simulink model "MMADC"  (R2021a)
settings: Solver=VariableStepAuto  StartTime=0.0  StopTime=1  RelTol=1e-3
values from neighbouring files (symbols this model uses):
  Cf = minimum_cap    [MMADC_main.m]
  clk_freq = 2.1*(nb_MAC+1)/nb_MAC*input_BW    (= 1684.375)    [MMADC_main.m]
  clk_period = 1/clk_freq    (= 0.000593692022263)    [MMADC_main.m]
  comparator_high_offset = 0.2*10e-4    (= 0.0002)    [MMADC_main.m]
  comparator_low_offset = -.1*10e-4    (= -0.0001)    [MMADC_main.m]
  comparator_noise_on = noise_on    (= 1)    [MMADC_main.m]
  comparator_noise_rms = 1*k*T* 2/3 / minimum_cap    [MMADC_main.m]
  comparator_offset_on = noise_on    (= 1)    [MMADC_main.m]
  k = 1.38064852e-23    [MMADC_main.m]
  LNA_bandwidth = 2.5*input_BW    (= 2000)    [MMADC_main.m]
  LNA_gain = 10^(36/20)*12*1.5849    (= 1200.00515432)    [MMADC_main.m]
  LNA_input_referred_noise = sqrt(pi/2*LNA_bandwidth*(194*10^-9)^2)    [MMADC_main.m]
  LNA_noise_on = noise_on    (= 1)    [MMADC_main.m]
  MM_incomplete_transfer_coeff = C1/(C1+C2)    [MMADC_main.m]
  MM_leakage_per_clk_cycle = 1    [MMADC_main.m]
  MM_sampling_noise = noise_on*((k*T * C1/(C1+C2)^2) + (k*T*(C1*C2/(C1+C2))/C2^2))    [MMADC_main.m]
  nb_MAC = 384    [MMADC_main.m]
  number_of_bits = 6    [MMADC_main.m]
  sample_time_jitter = 16e-12    (= 1.6e-11)    [MMADC_main.m]
  sampling_gain = Cs/Cf    [MMADC_main.m]
  sampling_jitter_on = noise_on    (= 1)    [MMADC_main.m]
  sensing_matrix = sensing_matrix_large(j:j+min(19,i-1),:)    [MMADC_main.m]
  sim_number = 0    [MMADC_main.m]
  switch_noise_on = noise_on    (= 1)    [MMADC_main.m]
  switching_noise = k*T/Cf    [MMADC_main.m]
  T = 293    [MMADC_main.m]
  Vref = 2    [MMADC_main.m]
  ZOH_delta = 0*Vref/(2^number_of_bits)    (= 0)    [MMADC_main.m]
libraries: simulink x100, simulink_extras x41, dspsigops x21, dspsrcs4 x21, spsFirstOrderFilterLib x1, dspswit3 x1
(part 6 of 10)

== system MMADC/Sensing Channel 8/SAR/ZOH+comparator ==
  Signal in : Inport
  DAC in : Inport  Port=2
  Input : Inport  Port=3
  Clk : Inport  Port=4
  AND{,1..3} (4 alike) : Logic  IconShape=distinctive  AllPortsSameDT=off  OutDataTypeStr=boolean
  Add : Sum  Inputs=+-
  Comparator : Subsystem  TreatAsAtomicUnit=on
      mask Display: text(.5, .5, 'Comparator', 'horizontalAlignment', 'center', 'verticalAlignment', 'middle')
  Compare To Constant : simulink/Logic and Bit Operations/Compare To Constant  relop===  const=2.0  OutDataTypeStr=boolean
  Constant : Constant  Value=ZOH_delta
  Count ZOH's : Subsystem
  D Latch : simulink_extras/Flip Flops/D Latch
      settings: SourceProductBaseCode=SL
  Delay : Delay
  Delay1 : Delay
  MATLAB Function : MATLAB Function  TreatAsAtomicUnit=on
  Multiport Switch : MultiPortSwitch
  Multiport Switch1 : MultiPortSwitch  Inputs=2  DiagnosticForDefault=None
  NOT1 : Logic  Operator=NOT  IconShape=distinctive  AllPortsSameDT=off  OutDataTypeStr=boolean
  OR1 : Logic  Operator=OR  IconShape=distinctive  AllPortsSameDT=off  OutDataTypeStr=boolean
  Old parallel ZOH comparator : Subsystem  Commented=on
      settings: PortSchema="{\"entries\":[{\"content\":{\"sides\":[{\"content\":{\"connectorIds\":[\"In1\",\"In2\"]},\"type\":\"ConnectorPlacement.EquallySpacedRectSide\",\"uuid\":\"06f7f8f5-dbcc-499c-adfd-56368a53e82b\"},{\"content\":{\"connectorIds\":[\"Out1\",\"Out2\"],\"side\":\"RIGHT\"},\"type\":\"ConnectorPlacement.EquallySpacedRectSide\",\"uuid\":\"5c800770-44b8-4ade-ac9f-191ddf2e034d\"},{\"content\":{\"connectorIds\":[\"In3\",\"In4\"],\"side\":\"TOP\"},\"type\":\"ConnectorPlacement.EquallySpacedRectSide\",\"uuid\":\"3f75a154-aff0-4c2f-90be-ad8d6219778d\"},{\"content\":{\"connectorIds\":[\"Out3\"],\"side\":\"BOTTOM\"},\"type\":\"ConnectorPlacement.EquallySpacedRectSide\",\"uuid\":\"1ea40a8b-dc4d-41fb-8cb2-c53fbb8e1a30\"},{\"content\":{\"connectorIds\":[],\"side\":\"HIDDEN\"},\"type\":\"ConnectorPlacement.EquallySpacedRectSide\",\"uuid\":\"dfb5a5fc-2880-46b8-8362-64f780de510f\"}]},\"type\":\"ConnectorPlacement.EquallySpacedConnector\",\"uuid\":\"ce700ed4-f915-4d6f-ac1f-aa4363807448\"}],\"packageUris\":[\"http://schema.mathworks.com/mf0/Connector/R2020b\"],\"version\":\"1.0\"}"
      mask Display: text(.5, .5, 'ZOH comparator', 'horizontalAlignment', 'center', 'verticalAlignment', 'middle')
  Subtract : Sum  Inputs=-+
  Output2 : Outport
  Output1 : Outport  Port=2
  Output : Outport  Port=3
  wires:
  Delay/1 -> Delay1/1, AND3/2
  Constant/1 -> Multiport Switch1/3
  DAC in/1 -> Multiport Switch/2, Subtract/2, Add/2
  D Latch/1 -> AND/1, Output1/1
  Add/1 -> Multiport Switch/3
  Signal in/1 -> Subtract/1, Add/1, Multiport Switch1/2
  Multiport Switch1/1 -> Comparator/1(y(t))
  Comparator/1(Comparator_out) -> Delay/1, AND2/2, Output2/1, NOT1/1
  Delay1/1 -> AND2/1
  MATLAB Function/1(y) -> Multiport Switch1/1, Multiport Switch/1
  Input/1 -> Compare To Constant/1, MATLAB Function/1(SAR_clk_cycle)
  Compare To Constant/1 -> AND1/1
  Count ZOH's/1(Out1) -> Output/1
  Multiport Switch/1 -> Comparator/2(DAC_in)
  OR1/1 -> D Latch/1
  Subtract/1 -> Multiport Switch/4
  NOT1/1 -> AND3/1
  AND3/1 -> OR1/2
  AND2/1 -> OR1/1
  AND/1 -> Count ZOH's/Trigger
  Clk/1 -> AND1/2
  AND1/1 -> D Latch/2, AND/2

== system MMADC/Sensing Channel 8/Sample&hold/Sample switch noise ==
  Input : Inport
  Trigger : TriggerPort  VariantControl=Variant
  Add1 : Sum
  Constant : Constant  Value=sampling_gain
  Constant1 : Constant  Value=0
  Constant2 : Constant  Value=switch_noise_on
  Multiply1 : Gain  Gain=sqrt(k*T/(sampling_gain*Cf))  OutDataTypeStr=Inherit: Same as input
  Product1 : Product
  Product2 : Product
  Random Number1 : RandomNumber  Variance=switching_noise
  Switch : Switch  Criteria=u2 > Threshold
  Zero-Order Hold1 : ZeroOrderHold  SampleTime=-1
  y(t) : Outport
  wires:
  Product2/1 -> y(t)/1
  Random Number1/1 -> Zero-Order Hold1/1
  Multiply1/1 -> Product1/1
  Add1/1 -> Product2/2
  Constant/1 -> Product2/1, Multiply1/1
  Constant2/1 -> Switch/2
  Constant1/1 -> Switch/3
  Product1/1 -> Switch/1
  Zero-Order Hold1/1 -> Product1/2
  Switch/1 -> Add1/1
  Input/1 -> Add1/2

== system MMADC/Sensing Channel 8/Sample&hold/Sample time jitter ==
  x(t) : Inport
  Add : Sum
  Constant : Constant  Value=sampling_jitter_on
  Derivative : Derivative
  Multiply : Gain  Gain=sample_time_jitter
  Product : Product
  Random Number : RandomNumber  SampleTime=clk_period*(number_of_bits+1)
  Switch : Switch  Criteria=u2 > Threshold
  Zero-Order Hold : ZeroOrderHold  SampleTime=-1
  Output : Outport
  wires:
  Random Number/1 -> Zero-Order Hold/1
  x(t)/1 -> Add/1, Switch/3, Derivative/1
  Zero-Order Hold/1 -> Multiply/1
  Product/1 -> Add/2
  Derivative/1 -> Product/1
  Multiply/1 -> Product/2
  Switch/1 -> Output/1
  Add/1 -> Switch/1
  Constant/1 -> Switch/2

== system MMADC/Sensing Channel 8/Subsystem2/Subsystem ==
  In1 : Inport
  In2 : Inport  Port=2
  Switch : Switch  Criteria=u2 ~= 0
  Zero : Constant  Value=0  OutDataTypeStr=Inherit: Inherit via back propagation
  Out1 : Outport
  wires:
  Switch/1 -> Out1/1
  In2/1 -> Switch/3
  In1/1 -> Switch/2
  Zero/1 -> Switch/1

== system MMADC/Sensing Channel 9/SAR/DAC ==
  NOB : Inport
  Vref : Inport  Port=2
  Input_code : Inport  Port=3
  DAC : MATLAB Function  TreatAsAtomicUnit=on
  y : Outport
  wires:
  NOB/1 -> DAC/2(number_of_bits)
  Vref/1 -> DAC/3(Vref)
  DAC/1(out) -> y/1
  Input_code/1 -> DAC/1(input_code)

== system MMADC/Sensing Channel 9/SAR/SAR ==
  Comparator_in : Inport  LatchByDelayingOutsideSignal=on
  ZOH : Inport  Port=2  LatchByDelayingOutsideSignal=on
  Number of bits : Inport  Port=3
  Trigger : TriggerPort  VariantControl=Variant
  SAR : MATLAB Function  TreatAsAtomicUnit=on
  Unit Delay : UnitDelay  SampleTime=-1  HasFrameUpgradeWarning=on
  Unit Delay1 : UnitDelay  SampleTime=-1  HasFrameUpgradeWarning=on
  Output : Outport
  SAR_done : Outport  Port=2  InitialOutput=0
  Output_code : Outport  Port=3  InitialOutput=zeros(number_of_bits, 1)
      settings: VarSizeSig=Yes
  wires:
  Number of bits/1 -> SAR/4(number_of_bits)
  Comparator_in/1 -> SAR/3(comparator_in)
  Unit Delay1/1 -> SAR/2(cycle_in)
  SAR/3(output_code) -> Output_code/1
  Unit Delay/1 -> SAR/1(input_code_decimal)
  SAR/1(output_code_decimal) -> Unit Delay/1
  SAR/4(done) -> SAR_done/1
  ZOH/1 -> SAR/5(ZOH_true)
  SAR/2(cycle_out) -> Output/1, Unit Delay1/1

== system MMADC/Sensing Channel 9/SAR/ZOH+comparator ==
  Signal in : Inport
  DAC in : Inport  Port=2
  Input : Inport  Port=3
  Clk : Inport  Port=4
  AND{,1..3} (4 alike) : Logic  IconShape=distinctive  AllPortsSameDT=off  OutDataTypeStr=boolean
  Add : Sum  Inputs=+-
  Comparator : Subsystem  TreatAsAtomicUnit=on
      mask Display: text(.5, .5, 'Comparator', 'horizontalAlignment', 'center', 'verticalAlignment', 'middle')
  Compare To Constant : simulink/Logic and Bit Operations/Compare To Constant  relop===  const=2.0  OutDataTypeStr=boolean
  Constant : Constant  Value=ZOH_delta
  Count ZOH's : Subsystem
  D Latch : simulink_extras/Flip Flops/D Latch
      settings: SourceProductBaseCode=SL
  Delay : Delay
  Delay1 : Delay
  MATLAB Function : MATLAB Function  TreatAsAtomicUnit=on
  Multiport Switch : MultiPortSwitch
  Multiport Switch1 : MultiPortSwitch  Inputs=2  DiagnosticForDefault=None
  NOT1 : Logic  Operator=NOT  IconShape=distinctive  AllPortsSameDT=off  OutDataTypeStr=boolean
  OR1 : Logic  Operator=OR  IconShape=distinctive  AllPortsSameDT=off  OutDataTypeStr=boolean
  Old parallel ZOH comparator : Subsystem  Commented=on
      settings: PortSchema="{\"entries\":[{\"content\":{\"sides\":[{\"content\":{\"connectorIds\":[\"In1\",\"In2\"]},\"type\":\"ConnectorPlacement.EquallySpacedRectSide\",\"uuid\":\"06f7f8f5-dbcc-499c-adfd-56368a53e82b\"},{\"content\":{\"connectorIds\":[\"Out1\",\"Out2\"],\"side\":\"RIGHT\"},\"type\":\"ConnectorPlacement.EquallySpacedRectSide\",\"uuid\":\"5c800770-44b8-4ade-ac9f-191ddf2e034d\"},{\"content\":{\"connectorIds\":[\"In3\",\"In4\"],\"side\":\"TOP\"},\"type\":\"ConnectorPlacement.EquallySpacedRectSide\",\"uuid\":\"3f75a154-aff0-4c2f-90be-ad8d6219778d\"},{\"content\":{\"connectorIds\":[\"Out3\"],\"side\":\"BOTTOM\"},\"type\":\"ConnectorPlacement.EquallySpacedRectSide\",\"uuid\":\"1ea40a8b-dc4d-41fb-8cb2-c53fbb8e1a30\"},{\"content\":{\"connectorIds\":[],\"side\":\"HIDDEN\"},\"type\":\"ConnectorPlacement.EquallySpacedRectSide\",\"uuid\":\"dfb5a5fc-2880-46b8-8362-64f780de510f\"}]},\"type\":\"ConnectorPlacement.EquallySpacedConnector\",\"uuid\":\"ce700ed4-f915-4d6f-ac1f-aa4363807448\"}],\"packageUris\":[\"http://schema.mathworks.com/mf0/Connector/R2020b\"],\"version\":\"1.0\"}"
      mask Display: text(.5, .5, 'ZOH comparator', 'horizontalAlignment', 'center', 'verticalAlignment', 'middle')
  Subtract : Sum  Inputs=-+
  Output2 : Outport
  Output1 : Outport  Port=2
  Output : Outport  Port=3
  wires:
  Delay/1 -> Delay1/1, AND3/2
  Constant/1 -> Multiport Switch1/3
  DAC in/1 -> Multiport Switch/2, Subtract/2, Add/2
  D Latch/1 -> AND/1, Output1/1
  Add/1 -> Multiport Switch/3
  Signal in/1 -> Subtract/1, Add/1, Multiport Switch1/2
  Multiport Switch1/1 -> Comparator/1(y(t))
  Comparator/1(Comparator_out) -> Delay/1, AND2/2, Output2/1, NOT1/1
  Delay1/1 -> AND2/1
  MATLAB Function/1(y) -> Multiport Switch1/1, Multiport Switch/1
  Input/1 -> Compare To Constant/1, MATLAB Function/1(SAR_clk_cycle)
  Compare To Constant/1 -> AND1/1
  Count ZOH's/1(Out1) -> Output/1
  Multiport Switch/1 -> Comparator/2(DAC_in)
  OR1/1 -> D Latch/1
  Subtract/1 -> Multiport Switch/4
  NOT1/1 -> AND3/1
  AND3/1 -> OR1/2
  AND2/1 -> OR1/1
  AND/1 -> Count ZOH's/Trigger
  Clk/1 -> AND1/2
  AND1/1 -> D Latch/2, AND/2

== system MMADC/Sensing Channel 9/Sample&hold/Sample switch noise ==
  Input : Inport
  Trigger : TriggerPort  VariantControl=Variant
  Add1 : Sum
  Constant : Constant  Value=sampling_gain
  Constant1 : Constant  Value=0
  Constant2 : Constant  Value=switch_noise_on
  Multiply1 : Gain  Gain=sqrt(k*T/(sampling_gain*Cf))  OutDataTypeStr=Inherit: Same as input
  Product1 : Product
  Product2 : Product
  Random Number1 : RandomNumber  Variance=switching_noise
  Switch : Switch  Criteria=u2 > Threshold
  Zero-Order Hold1 : ZeroOrderHold  SampleTime=-1
  y(t) : Outport
  wires:
  Product2/1 -> y(t)/1
  Random Number1/1 -> Zero-Order Hold1/1
  Multiply1/1 -> Product1/1
  Add1/1 -> Product2/2
  Constant/1 -> Product2/1, Multiply1/1
  Constant2/1 -> Switch/2
  Constant1/1 -> Switch/3
  Product1/1 -> Switch/1
  Zero-Order Hold1/1 -> Product1/2
  Switch/1 -> Add1/1
  Input/1 -> Add1/2

== system MMADC/Sensing Channel 9/Sample&hold/Sample time jitter ==
  x(t) : Inport
  Add : Sum
  Constant : Constant  Value=sampling_jitter_on
  Derivative : Derivative
  Multiply : Gain  Gain=sample_time_jitter
  Product : Product
  Random Number : RandomNumber  SampleTime=clk_period*(number_of_bits+1)
  Switch : Switch  Criteria=u2 > Threshold
  Zero-Order Hold : ZeroOrderHold  SampleTime=-1
  Output : Outport
  wires:
  Random Number/1 -> Zero-Order Hold/1
  x(t)/1 -> Add/1, Switch/3, Derivative/1
  Zero-Order Hold/1 -> Multiply/1
  Product/1 -> Add/2
  Derivative/1 -> Product/1
  Multiply/1 -> Product/2
  Switch/1 -> Output/1
  Add/1 -> Switch/1
  Constant/1 -> Switch/2

== system MMADC/Sensing Channel 9/Subsystem2/Subsystem ==
  In1 : Inport
  In2 : Inport  Port=2
  Switch : Switch  Criteria=u2 ~= 0
  Zero : Constant  Value=0  OutDataTypeStr=Inherit: Inherit via back propagation
  Out1 : Outport
  wires:
  Switch/1 -> Out1/1
  In2/1 -> Switch/3
  In1/1 -> Switch/2
  Zero/1 -> Switch/1

== system MMADC/Sensing Channel 1/SAR/ZOH+comparator/Comparator ==
  y(t) : Inport
  DAC_in : Inport  Port=2
  Add : Sum
  Add1 : Sum
  Compare To Zero : simulink/Logic and Bit Operations/Compare To Zero  relop=>  OutDataTypeStr=boolean
  Constant : Constant  Value=comparator_high_offset
  Constant1 : Constant  Value=comparator_low_offset
  Constant2 : Constant  Value=0
  Constant3 : Constant  Value=comparator_offset_on
  Constant4 : Constant  Value=0
  Constant5 : Constant  Value=comparator_noise_on
  Multiply : Gain  Gain=comparator_noise_rms
  Random Number : RandomNumber  Seed=sim_number  SampleTime=1/clk_freq
  Subtract : Sum  Inputs=+-
  Switch : Switch  Criteria=u2 > Threshold
  Switch1 : Switch  Criteria=u2 > Threshold
  Switch2 : Switch  Criteria=u2 > Threshold
  Unit Delay : UnitDelay  SampleTime=-1  HasFrameUpgradeWarning=on
  Comparator_out : Outport
  wires:
  Switch/1 -> Switch1/1
  Subtract/1 -> Add/1
  Constant/1 -> Switch/1
  Constant2/1 -> Switch1/3
  Add/1 -> Compare To Zero/1
  Switch1/1 -> Add/2
  Constant3/1 -> Switch1/2
  Unit Delay/1 -> Switch/2
  Constant1/1 -> Switch/3
  DAC_in/1 -> Subtract/2
  Add1/1 -> Subtract/1
  y(t)/1 -> Add1/2
  Random Number/1 -> Multiply/1
  Switch2/1 -> Add1/1
  Multiply/1 -> Switch2/1
  Constant4/1 -> Switch2/3
  Constant5/1 -> Switch2/2
  Compare To Zero/1 -> Unit Delay/1, Comparator_out/1

== system MMADC/Sensing Channel 1/SAR/ZOH+comparator/Count ZOH's ==
  Trigger : TriggerPort  VariantControl=Variant  PortDimensions=1
  Add : Sum  AccumDataTypeStr=double  OutDataTypeStr=double
  Constant : Constant
  Unit Delay : UnitDelay  SampleTime=-1  HasFrameUpgradeWarning=on
  Out1 : Outport
  wires:
  Constant/1 -> Add/1
  Add/1 -> Unit Delay/1, Out1/1
  Unit Delay/1 -> Add/2

== system MMADC/Sensing Channel 1/SAR/ZOH+comparator/Old parallel ZOH comparator ==
  Signal in : Inport
  DAC in : Inport  Port=2
  SAR done : Inport  Port=3
  Clk : Inport  Port=4
  " DAC-signal < delta?" : Subsystem  TreatAsAtomicUnit=on
      mask Display: text(.5, .5, 'Comparator', 'horizontalAlignment', 'center', 'verticalAlignment', 'middle')
  AND : Logic  IconShape=distinctive  AllPortsSameDT=off  OutDataTypeStr=boolean
  AND1 : Logic  IconShape=distinctive  AllPortsSameDT=off  OutDataTypeStr=boolean
  Add : Sum  Inputs=+-
  Constant : Constant  Value=ZOH_delta
  Count ZOH's : Subsystem
  D Latch : simulink_extras/Flip Flops/D Latch
      settings: SourceProductBaseCode=SL
  NOT : Logic  Operator=NOT  IconShape=distinctive  AllPortsSameDT=off  OutDataTypeStr=boolean
  OR : Logic  Operator=OR  IconShape=distinctive  AllPortsSameDT=off  OutDataTypeStr=boolean
  Signal-DAC < delta? : Subsystem  TreatAsAtomicUnit=on
      mask Display: text(.5, .5, 'Comparator', 'horizontalAlignment', 'center', 'verticalAlignment', 'middle')
  Signal>DAC? : Subsystem  TreatAsAtomicUnit=on
      mask Display: text(.5, .5, 'Comparator', 'horizontalAlignment', 'center', 'verticalAlignment', 'middle')
  Subtract : Sum  Inputs=-+
  Comparator_out : Outport
  Output1 : Outport  Port=2
  Output : Outport  Port=3
  wires:
  Signal>DAC?/1(Comparator_out) -> NOT/1, Comparator_out/1, AND1/1
  AND1/1 -> OR/1
  Subtract/1 -> " DAC-signal < delta?"/2(DAC_in)
  Signal in/1 -> Add/1, Subtract/1, Signal>DAC?/1(y(t))
  Clk/1 -> Signal>DAC?/Trigger, Signal-DAC < delta?/Trigger, " DAC-signal < delta?"/Trigger
  AND/1 -> OR/2
  " DAC-signal < delta?"/1(Comparator_out) -> AND/2  "comp2"
  Signal-DAC < delta?/1(Comparator_out) -> AND1/2  "comp1"
  Add/1 -> Signal-DAC < delta?/2(DAC_in)
  DAC in/1 -> Subtract/2, Add/2, Signal>DAC?/2(DAC_in)
  Constant/1 -> Signal-DAC < delta?/1(y(t)), " DAC-signal < delta?"/1(y(t))
  NOT/1 -> AND/1
  OR/1 -> D Latch/1
  D Latch/1 -> Count ZOH's/1(In1), Output1/1
  Count ZOH's/1(Out1) -> Output/1
  SAR done/1 -> Count ZOH's/Trigger, D Latch/2

== system MMADC/Sensing Channel 10/SAR/ZOH+comparator/Comparator ==
  y(t) : Inport
  DAC_in : Inport  Port=2
  Add : Sum
  Add1 : Sum
  Compare To Zero : simulink/Logic and Bit Operations/Compare To Zero  relop=>  OutDataTypeStr=boolean
  Constant : Constant  Value=comparator_high_offset
  Constant1 : Constant  Value=comparator_low_offset
  Constant2 : Constant  Value=0
  Constant3 : Constant  Value=comparator_offset_on
  Constant4 : Constant  Value=0
  Constant5 : Constant  Value=comparator_noise_on
  Multiply : Gain  Gain=comparator_noise_rms
  Random Number : RandomNumber  SampleTime=1/clk_freq
  Subtract : Sum  Inputs=+-
  Switch : Switch  Criteria=u2 > Threshold
  Switch1 : Switch  Criteria=u2 > Threshold
  Switch2 : Switch  Criteria=u2 > Threshold
  Unit Delay : UnitDelay  SampleTime=-1  HasFrameUpgradeWarning=on
  Comparator_out : Outport
  wires:
  Switch/1 -> Switch1/1
  Subtract/1 -> Add/1
  Constant/1 -> Switch/1
  Constant2/1 -> Switch1/3
  Add/1 -> Compare To Zero/1
  Switch1/1 -> Add/2
  Constant3/1 -> Switch1/2
  Unit Delay/1 -> Switch/2
  Constant1/1 -> Switch/3
  DAC_in/1 -> Subtract/2
  Add1/1 -> Subtract/1
  y(t)/1 -> Add1/2
  Random Number/1 -> Multiply/1
  Switch2/1 -> Add1/1
  Multiply/1 -> Switch2/1
  Constant4/1 -> Switch2/3
  Constant5/1 -> Switch2/2
  Compare To Zero/1 -> Unit Delay/1, Comparator_out/1

== system MMADC/Sensing Channel 10/SAR/ZOH+comparator/Count ZOH's ==
  Trigger : TriggerPort  VariantControl=Variant  PortDimensions=1
  Add : Sum  AccumDataTypeStr=double  OutDataTypeStr=double
  Constant : Constant
  Unit Delay : UnitDelay  SampleTime=-1  HasFrameUpgradeWarning=on
  Out1 : Outport
  wires:
  Constant/1 -> Add/1
  Add/1 -> Unit Delay/1, Out1/1
  Unit Delay/1 -> Add/2

== system MMADC/Sensing Channel 10/SAR/ZOH+comparator/Old parallel ZOH comparator ==
  Signal in : Inport
  DAC in : Inport  Port=2
  SAR done : Inport  Port=3
  Clk : Inport  Port=4
  " DAC-signal < delta?" : Subsystem  TreatAsAtomicUnit=on
      mask Display: text(.5, .5, 'Comparator', 'horizontalAlignment', 'center', 'verticalAlignment', 'middle')
  AND : Logic  IconShape=distinctive  AllPortsSameDT=off  OutDataTypeStr=boolean
  AND1 : Logic  IconShape=distinctive  AllPortsSameDT=off  OutDataTypeStr=boolean
  Add : Sum  Inputs=+-
  Constant : Constant  Value=ZOH_delta
  Count ZOH's : Subsystem
  D Latch : simulink_extras/Flip Flops/D Latch
      settings: SourceProductBaseCode=SL
  NOT : Logic  Operator=NOT  IconShape=distinctive  AllPortsSameDT=off  OutDataTypeStr=boolean
  OR : Logic  Operator=OR  IconShape=distinctive  AllPortsSameDT=off  OutDataTypeStr=boolean
  Signal-DAC < delta? : Subsystem  TreatAsAtomicUnit=on
      mask Display: text(.5, .5, 'Comparator', 'horizontalAlignment', 'center', 'verticalAlignment', 'middle')
  Signal>DAC? : Subsystem  TreatAsAtomicUnit=on
      mask Display: text(.5, .5, 'Comparator', 'horizontalAlignment', 'center', 'verticalAlignment', 'middle')
  Subtract : Sum  Inputs=-+
  Comparator_out : Outport
  Output1 : Outport  Port=2
  Output : Outport  Port=3
  wires:
  Signal>DAC?/1(Comparator_out) -> NOT/1, Comparator_out/1, AND1/1
  AND1/1 -> OR/1
  Subtract/1 -> " DAC-signal < delta?"/2(DAC_in)
  Signal in/1 -> Add/1, Subtract/1, Signal>DAC?/1(y(t))
  Clk/1 -> Signal>DAC?/Trigger, Signal-DAC < delta?/Trigger, " DAC-signal < delta?"/Trigger
  AND/1 -> OR/2
  " DAC-signal < delta?"/1(Comparator_out) -> AND/2  "comp2"
  Signal-DAC < delta?/1(Comparator_out) -> AND1/2  "comp1"
  Add/1 -> Signal-DAC < delta?/2(DAC_in)
  DAC in/1 -> Subtract/2, Add/2, Signal>DAC?/2(DAC_in)
  Constant/1 -> Signal-DAC < delta?/1(y(t)), " DAC-signal < delta?"/1(y(t))
  NOT/1 -> AND/1
  OR/1 -> D Latch/1
  D Latch/1 -> Count ZOH's/1(In1), Output1/1
  Count ZOH's/1(Out1) -> Output/1
  SAR done/1 -> Count ZOH's/Trigger, D Latch/2

== system MMADC/Sensing Channel 11/SAR/ZOH+comparator/Comparator ==
  y(t) : Inport
  DAC_in : Inport  Port=2
  Add : Sum
  Add1 : Sum
  Compare To Zero : simulink/Logic and Bit Operations/Compare To Zero  relop=>  OutDataTypeStr=boolean
  Constant : Constant  Value=comparator_high_offset
  Constant1 : Constant  Value=comparator_low_offset
  Constant2 : Constant  Value=0
  Constant3 : Constant  Value=comparator_offset_on
  Constant4 : Constant  Value=0
  Constant5 : Constant  Value=comparator_noise_on
  Multiply : Gain  Gain=comparator_noise_rms
  Random Number : RandomNumber  SampleTime=1/clk_freq
  Subtract : Sum  Inputs=+-
  Switch : Switch  Criteria=u2 > Threshold
  Switch1 : Switch  Criteria=u2 > Threshold
  Switch2 : Switch  Criteria=u2 > Threshold
  Unit Delay : UnitDelay  SampleTime=-1  HasFrameUpgradeWarning=on
  Comparator_out : Outport
  wires:
  Switch/1 -> Switch1/1
  Subtract/1 -> Add/1
  Constant/1 -> Switch/1
  Constant2/1 -> Switch1/3
  Add/1 -> Compare To Zero/1
  Switch1/1 -> Add/2
  Constant3/1 -> Switch1/2
  Unit Delay/1 -> Switch/2
  Constant1/1 -> Switch/3
  DAC_in/1 -> Subtract/2
  Add1/1 -> Subtract/1
  y(t)/1 -> Add1/2
  Random Number/1 -> Multiply/1
  Switch2/1 -> Add1/1
  Multiply/1 -> Switch2/1
  Constant4/1 -> Switch2/3
  Constant5/1 -> Switch2/2
  Compare To Zero/1 -> Unit Delay/1, Comparator_out/1

== system MMADC/Sensing Channel 11/SAR/ZOH+comparator/Count ZOH's ==
  Trigger : TriggerPort  VariantControl=Variant  PortDimensions=1
  Add : Sum  AccumDataTypeStr=double  OutDataTypeStr=double
  Constant : Constant
  Unit Delay : UnitDelay  SampleTime=-1  HasFrameUpgradeWarning=on
  Out1 : Outport
  wires:
  Constant/1 -> Add/1
  Add/1 -> Unit Delay/1, Out1/1
  Unit Delay/1 -> Add/2

== system MMADC/Sensing Channel 11/SAR/ZOH+comparator/Old parallel ZOH comparator ==
  Signal in : Inport
  DAC in : Inport  Port=2
  SAR done : Inport  Port=3
  Clk : Inport  Port=4
  " DAC-signal < delta?" : Subsystem  TreatAsAtomicUnit=on
      mask Display: text(.5, .5, 'Comparator', 'horizontalAlignment', 'center', 'verticalAlignment', 'middle')
  AND : Logic  IconShape=distinctive  AllPortsSameDT=off  OutDataTypeStr=boolean
  AND1 : Logic  IconShape=distinctive  AllPortsSameDT=off  OutDataTypeStr=boolean
  Add : Sum  Inputs=+-
  Constant : Constant  Value=ZOH_delta
  Count ZOH's : Subsystem
  D Latch : simulink_extras/Flip Flops/D Latch
      settings: SourceProductBaseCode=SL
  NOT : Logic  Operator=NOT  IconShape=distinctive  AllPortsSameDT=off  OutDataTypeStr=boolean
  OR : Logic  Operator=OR  IconShape=distinctive  AllPortsSameDT=off  OutDataTypeStr=boolean
  Signal-DAC < delta? : Subsystem  TreatAsAtomicUnit=on
      mask Display: text(.5, .5, 'Comparator', 'horizontalAlignment', 'center', 'verticalAlignment', 'middle')
  Signal>DAC? : Subsystem  TreatAsAtomicUnit=on
      mask Display: text(.5, .5, 'Comparator', 'horizontalAlignment', 'center', 'verticalAlignment', 'middle')
  Subtract : Sum  Inputs=-+
  Comparator_out : Outport
  Output1 : Outport  Port=2
  Output : Outport  Port=3
  wires:
  Signal>DAC?/1(Comparator_out) -> NOT/1, Comparator_out/1, AND1/1
  AND1/1 -> OR/1
  Subtract/1 -> " DAC-signal < delta?"/2(DAC_in)
  Signal in/1 -> Add/1, Subtract/1, Signal>DAC?/1(y(t))
  Clk/1 -> Signal>DAC?/Trigger, Signal-DAC < delta?/Trigger, " DAC-signal < delta?"/Trigger
  AND/1 -> OR/2
  " DAC-signal < delta?"/1(Comparator_out) -> AND/2  "comp2"
  Signal-DAC < delta?/1(Comparator_out) -> AND1/2  "comp1"
  Add/1 -> Signal-DAC < delta?/2(DAC_in)
  DAC in/1 -> Subtract/2, Add/2, Signal>DAC?/2(DAC_in)
  Constant/1 -> Signal-DAC < delta?/1(y(t)), " DAC-signal < delta?"/1(y(t))
  NOT/1 -> AND/1
  OR/1 -> D Latch/1
  D Latch/1 -> Count ZOH's/1(In1), Output1/1
  Count ZOH's/1(Out1) -> Output/1
  SAR done/1 -> Count ZOH's/Trigger, D Latch/2

== system MMADC/Sensing Channel 12/SAR/ZOH+comparator/Comparator ==
  y(t) : Inport
  DAC_in : Inport  Port=2
  Add : Sum
  Add1 : Sum
  Compare To Zero : simulink/Logic and Bit Operations/Compare To Zero  relop=>  OutDataTypeStr=boolean
  Constant : Constant  Value=comparator_high_offset
  Constant1 : Constant  Value=comparator_low_offset
  Constant2 : Constant  Value=0
  Constant3 : Constant  Value=comparator_offset_on
  Constant4 : Constant  Value=0
  Constant5 : Constant  Value=comparator_noise_on
  Multiply : Gain  Gain=comparator_noise_rms
  Random Number : RandomNumber  SampleTime=1/clk_freq
  Subtract : Sum  Inputs=+-
  Switch : Switch  Criteria=u2 > Threshold
  Switch1 : Switch  Criteria=u2 > Threshold
  Switch2 : Switch  Criteria=u2 > Threshold
  Unit Delay : UnitDelay  SampleTime=-1  HasFrameUpgradeWarning=on
  Comparator_out : Outport
  wires:
  Switch/1 -> Switch1/1
  Subtract/1 -> Add/1
  Constant/1 -> Switch/1
  Constant2/1 -> Switch1/3
  Add/1 -> Compare To Zero/1
  Switch1/1 -> Add/2
  Constant3/1 -> Switch1/2
  Unit Delay/1 -> Switch/2
  Constant1/1 -> Switch/3
  DAC_in/1 -> Subtract/2
  Add1/1 -> Subtract/1
  y(t)/1 -> Add1/2
  Random Number/1 -> Multiply/1
  Switch2/1 -> Add1/1
  Multiply/1 -> Switch2/1
  Constant4/1 -> Switch2/3
  Constant5/1 -> Switch2/2
  Compare To Zero/1 -> Unit Delay/1, Comparator_out/1

== system MMADC/Sensing Channel 12/SAR/ZOH+comparator/Count ZOH's ==
  Trigger : TriggerPort  VariantControl=Variant  PortDimensions=1
  Add : Sum  AccumDataTypeStr=double  OutDataTypeStr=double
  Constant : Constant
  Unit Delay : UnitDelay  SampleTime=-1  HasFrameUpgradeWarning=on
  Out1 : Outport
  wires:
  Constant/1 -> Add/1
  Add/1 -> Unit Delay/1, Out1/1
  Unit Delay/1 -> Add/2

== system MMADC/Sensing Channel 12/SAR/ZOH+comparator/Old parallel ZOH comparator ==
  Signal in : Inport
  DAC in : Inport  Port=2
  SAR done : Inport  Port=3
  Clk : Inport  Port=4
  " DAC-signal < delta?" : Subsystem  TreatAsAtomicUnit=on
      mask Display: text(.5, .5, 'Comparator', 'horizontalAlignment', 'center', 'verticalAlignment', 'middle')
  AND : Logic  IconShape=distinctive  AllPortsSameDT=off  OutDataTypeStr=boolean
  AND1 : Logic  IconShape=distinctive  AllPortsSameDT=off  OutDataTypeStr=boolean
  Add : Sum  Inputs=+-
  Constant : Constant  Value=ZOH_delta
  Count ZOH's : Subsystem
  D Latch : simulink_extras/Flip Flops/D Latch
      settings: SourceProductBaseCode=SL
  NOT : Logic  Operator=NOT  IconShape=distinctive  AllPortsSameDT=off  OutDataTypeStr=boolean
  OR : Logic  Operator=OR  IconShape=distinctive  AllPortsSameDT=off  OutDataTypeStr=boolean
  Signal-DAC < delta? : Subsystem  TreatAsAtomicUnit=on
      mask Display: text(.5, .5, 'Comparator', 'horizontalAlignment', 'center', 'verticalAlignment', 'middle')
  Signal>DAC? : Subsystem  TreatAsAtomicUnit=on
      mask Display: text(.5, .5, 'Comparator', 'horizontalAlignment', 'center', 'verticalAlignment', 'middle')
  Subtract : Sum  Inputs=-+
  Comparator_out : Outport
  Output1 : Outport  Port=2
  Output : Outport  Port=3
  wires:
  Signal>DAC?/1(Comparator_out) -> NOT/1, Comparator_out/1, AND1/1
  AND1/1 -> OR/1
  Subtract/1 -> " DAC-signal < delta?"/2(DAC_in)
  Signal in/1 -> Add/1, Subtract/1, Signal>DAC?/1(y(t))
  Clk/1 -> Signal>DAC?/Trigger, Signal-DAC < delta?/Trigger, " DAC-signal < delta?"/Trigger
  AND/1 -> OR/2
  " DAC-signal < delta?"/1(Comparator_out) -> AND/2  "comp2"
  Signal-DAC < delta?/1(Comparator_out) -> AND1/2  "comp1"
  Add/1 -> Signal-DAC < delta?/2(DAC_in)
  DAC in/1 -> Subtract/2, Add/2, Signal>DAC?/2(DAC_in)
  Constant/1 -> Signal-DAC < delta?/1(y(t)), " DAC-signal < delta?"/1(y(t))
  NOT/1 -> AND/1
  OR/1 -> D Latch/1
  D Latch/1 -> Count ZOH's/1(In1), Output1/1
  Count ZOH's/1(Out1) -> Output/1
  SAR done/1 -> Count ZOH's/Trigger, D Latch/2

== system MMADC/Sensing Channel 13/SAR/ZOH+comparator/Comparator ==
  y(t) : Inport
  DAC_in : Inport  Port=2
  Add : Sum
  Add1 : Sum
  Compare To Zero : simulink/Logic and Bit Operations/Compare To Zero  relop=>  OutDataTypeStr=boolean
  Constant : Constant  Value=comparator_high_offset
  Constant1 : Constant  Value=comparator_low_offset
  Constant2 : Constant  Value=0
  Constant3 : Constant  Value=comparator_offset_on
  Constant4 : Constant  Value=0
  Constant5 : Constant  Value=comparator_noise_on
  Multiply : Gain  Gain=comparator_noise_rms
  Random Number : RandomNumber  SampleTime=1/clk_freq
  Subtract : Sum  Inputs=+-
  Switch : Switch  Criteria=u2 > Threshold
  Switch1 : Switch  Criteria=u2 > Threshold
  Switch2 : Switch  Criteria=u2 > Threshold
  Unit Delay : UnitDelay  SampleTime=-1  HasFrameUpgradeWarning=on
  Comparator_out : Outport
  wires:
  Switch/1 -> Switch1/1
  Subtract/1 -> Add/1
  Constant/1 -> Switch/1
  Constant2/1 -> Switch1/3
  Add/1 -> Compare To Zero/1
  Switch1/1 -> Add/2
  Constant3/1 -> Switch1/2
  Unit Delay/1 -> Switch/2
  Constant1/1 -> Switch/3
  DAC_in/1 -> Subtract/2
  Add1/1 -> Subtract/1
  y(t)/1 -> Add1/2
  Random Number/1 -> Multiply/1
  Switch2/1 -> Add1/1
  Multiply/1 -> Switch2/1
  Constant4/1 -> Switch2/3
  Constant5/1 -> Switch2/2
  Compare To Zero/1 -> Unit Delay/1, Comparator_out/1

== system MMADC/Sensing Channel 13/SAR/ZOH+comparator/Count ZOH's ==
  Trigger : TriggerPort  VariantControl=Variant  PortDimensions=1
  Add : Sum  AccumDataTypeStr=double  OutDataTypeStr=double
  Constant : Constant
  Unit Delay : UnitDelay  SampleTime=-1  HasFrameUpgradeWarning=on
  Out1 : Outport
  wires:
  Constant/1 -> Add/1
  Add/1 -> Unit Delay/1, Out1/1
  Unit Delay/1 -> Add/2

== system MMADC/Sensing Channel 13/SAR/ZOH+comparator/Old parallel ZOH comparator ==
  Signal in : Inport
  DAC in : Inport  Port=2
  SAR done : Inport  Port=3
  Clk : Inport  Port=4
  " DAC-signal < delta?" : Subsystem  TreatAsAtomicUnit=on
      mask Display: text(.5, .5, 'Comparator', 'horizontalAlignment', 'center', 'verticalAlignment', 'middle')
  AND : Logic  IconShape=distinctive  AllPortsSameDT=off  OutDataTypeStr=boolean
  AND1 : Logic  IconShape=distinctive  AllPortsSameDT=off  OutDataTypeStr=boolean
  Add : Sum  Inputs=+-
  Constant : Constant  Value=ZOH_delta
  Count ZOH's : Subsystem
  D Latch : simulink_extras/Flip Flops/D Latch
      settings: SourceProductBaseCode=SL
  NOT : Logic  Operator=NOT  IconShape=distinctive  AllPortsSameDT=off  OutDataTypeStr=boolean
  OR : Logic  Operator=OR  IconShape=distinctive  AllPortsSameDT=off  OutDataTypeStr=boolean
  Signal-DAC < delta? : Subsystem  TreatAsAtomicUnit=on
      mask Display: text(.5, .5, 'Comparator', 'horizontalAlignment', 'center', 'verticalAlignment', 'middle')
  Signal>DAC? : Subsystem  TreatAsAtomicUnit=on
      mask Display: text(.5, .5, 'Comparator', 'horizontalAlignment', 'center', 'verticalAlignment', 'middle')
  Subtract : Sum  Inputs=-+
  Comparator_out : Outport
  Output1 : Outport  Port=2
  Output : Outport  Port=3
  wires:
  Signal>DAC?/1(Comparator_out) -> NOT/1, Comparator_out/1, AND1/1
  AND1/1 -> OR/1
  Subtract/1 -> " DAC-signal < delta?"/2(DAC_in)
  Signal in/1 -> Add/1, Subtract/1, Signal>DAC?/1(y(t))
  Clk/1 -> Signal>DAC?/Trigger, Signal-DAC < delta?/Trigger, " DAC-signal < delta?"/Trigger
  AND/1 -> OR/2
  " DAC-signal < delta?"/1(Comparator_out) -> AND/2  "comp2"
  Signal-DAC < delta?/1(Comparator_out) -> AND1/2  "comp1"
  Add/1 -> Signal-DAC < delta?/2(DAC_in)
  DAC in/1 -> Subtract/2, Add/2, Signal>DAC?/2(DAC_in)
  Constant/1 -> Signal-DAC < delta?/1(y(t)), " DAC-signal < delta?"/1(y(t))
  NOT/1 -> AND/1
  OR/1 -> D Latch/1
  D Latch/1 -> Count ZOH's/1(In1), Output1/1
  Count ZOH's/1(Out1) -> Output/1
  SAR done/1 -> Count ZOH's/Trigger, D Latch/2

== system MMADC/Sensing Channel 14/SAR/ZOH+comparator/Comparator ==
  y(t) : Inport
  DAC_in : Inport  Port=2
  Add : Sum
  Add1 : Sum
  Compare To Zero : simulink/Logic and Bit Operations/Compare To Zero  relop=>  OutDataTypeStr=boolean
  Constant : Constant  Value=comparator_high_offset
  Constant1 : Constant  Value=comparator_low_offset
  Constant2 : Constant  Value=0
  Constant3 : Constant  Value=comparator_offset_on
  Constant4 : Constant  Value=0
  Constant5 : Constant  Value=comparator_noise_on
  Multiply : Gain  Gain=comparator_noise_rms
  Random Number : RandomNumber  SampleTime=1/clk_freq
  Subtract : Sum  Inputs=+-
  Switch : Switch  Criteria=u2 > Threshold
  Switch1 : Switch  Criteria=u2 > Threshold
  Switch2 : Switch  Criteria=u2 > Threshold
  Unit Delay : UnitDelay  SampleTime=-1  HasFrameUpgradeWarning=on
  Comparator_out : Outport
  wires:
  Switch/1 -> Switch1/1
  Subtract/1 -> Add/1
  Constant/1 -> Switch/1
  Constant2/1 -> Switch1/3
  Add/1 -> Compare To Zero/1
  Switch1/1 -> Add/2
  Constant3/1 -> Switch1/2
  Unit Delay/1 -> Switch/2
  Constant1/1 -> Switch/3
  DAC_in/1 -> Subtract/2
  Add1/1 -> Subtract/1
  y(t)/1 -> Add1/2
  Random Number/1 -> Multiply/1
  Switch2/1 -> Add1/1
  Multiply/1 -> Switch2/1
  Constant4/1 -> Switch2/3
  Constant5/1 -> Switch2/2
  Compare To Zero/1 -> Unit Delay/1, Comparator_out/1

== system MMADC/Sensing Channel 14/SAR/ZOH+comparator/Count ZOH's ==
  Trigger : TriggerPort  VariantControl=Variant  PortDimensions=1
  Add : Sum  AccumDataTypeStr=double  OutDataTypeStr=double
  Constant : Constant
  Unit Delay : UnitDelay  SampleTime=-1  HasFrameUpgradeWarning=on
  Out1 : Outport
  wires:
  Constant/1 -> Add/1
  Add/1 -> Unit Delay/1, Out1/1
  Unit Delay/1 -> Add/2

== system MMADC/Sensing Channel 14/SAR/ZOH+comparator/Old parallel ZOH comparator ==
  Signal in : Inport
  DAC in : Inport  Port=2
  SAR done : Inport  Port=3
  Clk : Inport  Port=4
  " DAC-signal < delta?" : Subsystem  TreatAsAtomicUnit=on
      mask Display: text(.5, .5, 'Comparator', 'horizontalAlignment', 'center', 'verticalAlignment', 'middle')
  AND : Logic  IconShape=distinctive  AllPortsSameDT=off  OutDataTypeStr=boolean
  AND1 : Logic  IconShape=distinctive  AllPortsSameDT=off  OutDataTypeStr=boolean
  Add : Sum  Inputs=+-
  Constant : Constant  Value=ZOH_delta
  Count ZOH's : Subsystem
  D Latch : simulink_extras/Flip Flops/D Latch
      settings: SourceProductBaseCode=SL
  NOT : Logic  Operator=NOT  IconShape=distinctive  AllPortsSameDT=off  OutDataTypeStr=boolean
  OR : Logic  Operator=OR  IconShape=distinctive  AllPortsSameDT=off  OutDataTypeStr=boolean
  Signal-DAC < delta? : Subsystem  TreatAsAtomicUnit=on
      mask Display: text(.5, .5, 'Comparator', 'horizontalAlignment', 'center', 'verticalAlignment', 'middle')
  Signal>DAC? : Subsystem  TreatAsAtomicUnit=on
      mask Display: text(.5, .5, 'Comparator', 'horizontalAlignment', 'center', 'verticalAlignment', 'middle')
  Subtract : Sum  Inputs=-+
  Comparator_out : Outport
  Output1 : Outport  Port=2
  Output : Outport  Port=3
  wires:
  Signal>DAC?/1(Comparator_out) -> NOT/1, Comparator_out/1, AND1/1
  AND1/1 -> OR/1
  Subtract/1 -> " DAC-signal < delta?"/2(DAC_in)
  Signal in/1 -> Add/1, Subtract/1, Signal>DAC?/1(y(t))
  Clk/1 -> Signal>DAC?/Trigger, Signal-DAC < delta?/Trigger, " DAC-signal < delta?"/Trigger
  AND/1 -> OR/2
  " DAC-signal < delta?"/1(Comparator_out) -> AND/2  "comp2"
  Signal-DAC < delta?/1(Comparator_out) -> AND1/2  "comp1"
  Add/1 -> Signal-DAC < delta?/2(DAC_in)
  DAC in/1 -> Subtract/2, Add/2, Signal>DAC?/2(DAC_in)
  Constant/1 -> Signal-DAC < delta?/1(y(t)), " DAC-signal < delta?"/1(y(t))
  NOT/1 -> AND/1
  OR/1 -> D Latch/1
  D Latch/1 -> Count ZOH's/1(In1), Output1/1
  Count ZOH's/1(Out1) -> Output/1
  SAR done/1 -> Count ZOH's/Trigger, D Latch/2

== system MMADC/Sensing Channel 15/SAR/ZOH+comparator/Comparator ==
  y(t) : Inport
  DAC_in : Inport  Port=2
  Add : Sum
  Add1 : Sum
  Compare To Zero : simulink/Logic and Bit Operations/Compare To Zero  relop=>  OutDataTypeStr=boolean
  Constant : Constant  Value=comparator_high_offset
  Constant1 : Constant  Value=comparator_low_offset
  Constant2 : Constant  Value=0
  Constant3 : Constant  Value=comparator_offset_on
  Constant4 : Constant  Value=0
  Constant5 : Constant  Value=comparator_noise_on
  Multiply : Gain  Gain=comparator_noise_rms
  Random Number : RandomNumber  SampleTime=1/clk_freq
  Subtract : Sum  Inputs=+-
  Switch : Switch  Criteria=u2 > Threshold
  Switch1 : Switch  Criteria=u2 > Threshold
  Switch2 : Switch  Criteria=u2 > Threshold
  Unit Delay : UnitDelay  SampleTime=-1  HasFrameUpgradeWarning=on
  Comparator_out : Outport
  wires:
  Switch/1 -> Switch1/1
  Subtract/1 -> Add/1
  Constant/1 -> Switch/1
  Constant2/1 -> Switch1/3
  Add/1 -> Compare To Zero/1
  Switch1/1 -> Add/2
  Constant3/1 -> Switch1/2
  Unit Delay/1 -> Switch/2
  Constant1/1 -> Switch/3
  DAC_in/1 -> Subtract/2
  Add1/1 -> Subtract/1
  y(t)/1 -> Add1/2
  Random Number/1 -> Multiply/1
  Switch2/1 -> Add1/1
  Multiply/1 -> Switch2/1
  Constant4/1 -> Switch2/3
  Constant5/1 -> Switch2/2
  Compare To Zero/1 -> Unit Delay/1, Comparator_out/1

== system MMADC/Sensing Channel 15/SAR/ZOH+comparator/Count ZOH's ==
  Trigger : TriggerPort  VariantControl=Variant  PortDimensions=1
  Add : Sum  AccumDataTypeStr=double  OutDataTypeStr=double
  Constant : Constant
  Unit Delay : UnitDelay  SampleTime=-1  HasFrameUpgradeWarning=on
  Out1 : Outport
  wires:
  Constant/1 -> Add/1
  Add/1 -> Unit Delay/1, Out1/1
  Unit Delay/1 -> Add/2

== system MMADC/Sensing Channel 15/SAR/ZOH+comparator/Old parallel ZOH comparator ==
  Signal in : Inport
  DAC in : Inport  Port=2
  SAR done : Inport  Port=3
  Clk : Inport  Port=4
  " DAC-signal < delta?" : Subsystem  TreatAsAtomicUnit=on
      mask Display: text(.5, .5, 'Comparator', 'horizontalAlignment', 'center', 'verticalAlignment', 'middle')
  AND : Logic  IconShape=distinctive  AllPortsSameDT=off  OutDataTypeStr=boolean
  AND1 : Logic  IconShape=distinctive  AllPortsSameDT=off  OutDataTypeStr=boolean
  Add : Sum  Inputs=+-
  Constant : Constant  Value=ZOH_delta
  Count ZOH's : Subsystem
  D Latch : simulink_extras/Flip Flops/D Latch
      settings: SourceProductBaseCode=SL
  NOT : Logic  Operator=NOT  IconShape=distinctive  AllPortsSameDT=off  OutDataTypeStr=boolean
  OR : Logic  Operator=OR  IconShape=distinctive  AllPortsSameDT=off  OutDataTypeStr=boolean
  Signal-DAC < delta? : Subsystem  TreatAsAtomicUnit=on
      mask Display: text(.5, .5, 'Comparator', 'horizontalAlignment', 'center', 'verticalAlignment', 'middle')
  Signal>DAC? : Subsystem  TreatAsAtomicUnit=on
      mask Display: text(.5, .5, 'Comparator', 'horizontalAlignment', 'center', 'verticalAlignment', 'middle')
  Subtract : Sum  Inputs=-+
  Comparator_out : Outport
  Output1 : Outport  Port=2
  Output : Outport  Port=3
  wires:
  Signal>DAC?/1(Comparator_out) -> NOT/1, Comparator_out/1, AND1/1
  AND1/1 -> OR/1
  Subtract/1 -> " DAC-signal < delta?"/2(DAC_in)
  Signal in/1 -> Add/1, Subtract/1, Signal>DAC?/1(y(t))
  Clk/1 -> Signal>DAC?/Trigger, Signal-DAC < delta?/Trigger, " DAC-signal < delta?"/Trigger
  AND/1 -> OR/2
  " DAC-signal < delta?"/1(Comparator_out) -> AND/2  "comp2"
  Signal-DAC < delta?/1(Comparator_out) -> AND1/2  "comp1"
  Add/1 -> Signal-DAC < delta?/2(DAC_in)
  DAC in/1 -> Subtract/2, Add/2, Signal>DAC?/2(DAC_in)
  Constant/1 -> Signal-DAC < delta?/1(y(t)), " DAC-signal < delta?"/1(y(t))
  NOT/1 -> AND/1
  OR/1 -> D Latch/1
  D Latch/1 -> Count ZOH's/1(In1), Output1/1
  Count ZOH's/1(Out1) -> Output/1
  SAR done/1 -> Count ZOH's/Trigger, D Latch/2

== system MMADC/Sensing Channel 16/SAR/ZOH+comparator/Comparator ==
  y(t) : Inport
  DAC_in : Inport  Port=2
  Add : Sum
  Add1 : Sum
  Compare To Zero : simulink/Logic and Bit Operations/Compare To Zero  relop=>  OutDataTypeStr=boolean
  Constant : Constant  Value=comparator_high_offset
  Constant1 : Constant  Value=comparator_low_offset
  Constant2 : Constant  Value=0
  Constant3 : Constant  Value=comparator_offset_on
  Constant4 : Constant  Value=0
  Constant5 : Constant  Value=comparator_noise_on
  Multiply : Gain  Gain=comparator_noise_rms
  Random Number : RandomNumber  SampleTime=1/clk_freq
  Subtract : Sum  Inputs=+-
  Switch : Switch  Criteria=u2 > Threshold
  Switch1 : Switch  Criteria=u2 > Threshold
  Switch2 : Switch  Criteria=u2 > Threshold
  Unit Delay : UnitDelay  SampleTime=-1  HasFrameUpgradeWarning=on
  Comparator_out : Outport
  wires:
  Switch/1 -> Switch1/1
  Subtract/1 -> Add/1
  Constant/1 -> Switch/1
  Constant2/1 -> Switch1/3
  Add/1 -> Compare To Zero/1
  Switch1/1 -> Add/2
  Constant3/1 -> Switch1/2
  Unit Delay/1 -> Switch/2
  Constant1/1 -> Switch/3
  DAC_in/1 -> Subtract/2
  Add1/1 -> Subtract/1
  y(t)/1 -> Add1/2
  Random Number/1 -> Multiply/1
  Switch2/1 -> Add1/1
  Multiply/1 -> Switch2/1
  Constant4/1 -> Switch2/3
  Constant5/1 -> Switch2/2
  Compare To Zero/1 -> Unit Delay/1, Comparator_out/1

== system MMADC/Sensing Channel 16/SAR/ZOH+comparator/Count ZOH's ==
  Trigger : TriggerPort  VariantControl=Variant  PortDimensions=1
  Add : Sum  AccumDataTypeStr=double  OutDataTypeStr=double
  Constant : Constant
  Unit Delay : UnitDelay  SampleTime=-1  HasFrameUpgradeWarning=on
  Out1 : Outport
  wires:
  Constant/1 -> Add/1
  Add/1 -> Unit Delay/1, Out1/1
  Unit Delay/1 -> Add/2

== system MMADC/Sensing Channel 16/SAR/ZOH+comparator/Old parallel ZOH comparator ==
  Signal in : Inport
  DAC in : Inport  Port=2
  SAR done : Inport  Port=3
  Clk : Inport  Port=4
  " DAC-signal < delta?" : Subsystem  TreatAsAtomicUnit=on
      mask Display: text(.5, .5, 'Comparator', 'horizontalAlignment', 'center', 'verticalAlignment', 'middle')
  AND : Logic  IconShape=distinctive  AllPortsSameDT=off  OutDataTypeStr=boolean
  AND1 : Logic  IconShape=distinctive  AllPortsSameDT=off  OutDataTypeStr=boolean
  Add : Sum  Inputs=+-
  Constant : Constant  Value=ZOH_delta
  Count ZOH's : Subsystem
  D Latch : simulink_extras/Flip Flops/D Latch
      settings: SourceProductBaseCode=SL
  NOT : Logic  Operator=NOT  IconShape=distinctive  AllPortsSameDT=off  OutDataTypeStr=boolean
  OR : Logic  Operator=OR  IconShape=distinctive  AllPortsSameDT=off  OutDataTypeStr=boolean
  Signal-DAC < delta? : Subsystem  TreatAsAtomicUnit=on
      mask Display: text(.5, .5, 'Comparator', 'horizontalAlignment', 'center', 'verticalAlignment', 'middle')
  Signal>DAC? : Subsystem  TreatAsAtomicUnit=on
      mask Display: text(.5, .5, 'Comparator', 'horizontalAlignment', 'center', 'verticalAlignment', 'middle')
  Subtract : Sum  Inputs=-+
  Comparator_out : Outport
  Output1 : Outport  Port=2
  Output : Outport  Port=3
  wires:
  Signal>DAC?/1(Comparator_out) -> NOT/1, Comparator_out/1, AND1/1
  AND1/1 -> OR/1
  Subtract/1 -> " DAC-signal < delta?"/2(DAC_in)
  Signal in/1 -> Add/1, Subtract/1, Signal>DAC?/1(y(t))
  Clk/1 -> Signal>DAC?/Trigger, Signal-DAC < delta?/Trigger, " DAC-signal < delta?"/Trigger
  AND/1 -> OR/2
  " DAC-signal < delta?"/1(Comparator_out) -> AND/2  "comp2"
  Signal-DAC < delta?/1(Comparator_out) -> AND1/2  "comp1"
  Add/1 -> Signal-DAC < delta?/2(DAC_in)
  DAC in/1 -> Subtract/2, Add/2, Signal>DAC?/2(DAC_in)
  Constant/1 -> Signal-DAC < delta?/1(y(t)), " DAC-signal < delta?"/1(y(t))
  NOT/1 -> AND/1
  OR/1 -> D Latch/1
  D Latch/1 -> Count ZOH's/1(In1), Output1/1
  Count ZOH's/1(Out1) -> Output/1
  SAR done/1 -> Count ZOH's/Trigger, D Latch/2

== system MMADC/Sensing Channel 17/SAR/ZOH+comparator/Comparator ==
  y(t) : Inport
  DAC_in : Inport  Port=2
  Add : Sum
  Add1 : Sum
  Compare To Zero : simulink/Logic and Bit Operations/Compare To Zero  relop=>  OutDataTypeStr=boolean
  Constant : Constant  Value=comparator_high_offset
  Constant1 : Constant  Value=comparator_low_offset
  Constant2 : Constant  Value=0
  Constant3 : Constant  Value=comparator_offset_on
  Constant4 : Constant  Value=0
  Constant5 : Constant  Value=comparator_noise_on
  Multiply : Gain  Gain=comparator_noise_rms
  Random Number : RandomNumber  SampleTime=1/clk_freq
  Subtract : Sum  Inputs=+-
  Switch : Switch  Criteria=u2 > Threshold
  Switch1 : Switch  Criteria=u2 > Threshold
  Switch2 : Switch  Criteria=u2 > Threshold
  Unit Delay : UnitDelay  SampleTime=-1  HasFrameUpgradeWarning=on
  Comparator_out : Outport
  wires:
  Switch/1 -> Switch1/1
  Subtract/1 -> Add/1
  Constant/1 -> Switch/1
  Constant2/1 -> Switch1/3
  Add/1 -> Compare To Zero/1
  Switch1/1 -> Add/2
  Constant3/1 -> Switch1/2
  Unit Delay/1 -> Switch/2
  Constant1/1 -> Switch/3
  DAC_in/1 -> Subtract/2
  Add1/1 -> Subtract/1
  y(t)/1 -> Add1/2
  Random Number/1 -> Multiply/1
  Switch2/1 -> Add1/1
  Multiply/1 -> Switch2/1
  Constant4/1 -> Switch2/3
  Constant5/1 -> Switch2/2
  Compare To Zero/1 -> Unit Delay/1, Comparator_out/1

== system MMADC/Sensing Channel 17/SAR/ZOH+comparator/Count ZOH's ==
  Trigger : TriggerPort  VariantControl=Variant  PortDimensions=1
  Add : Sum  AccumDataTypeStr=double  OutDataTypeStr=double
  Constant : Constant
  Unit Delay : UnitDelay  SampleTime=-1  HasFrameUpgradeWarning=on
  Out1 : Outport
  wires:
  Constant/1 -> Add/1
  Add/1 -> Unit Delay/1, Out1/1
  Unit Delay/1 -> Add/2

== system MMADC/Sensing Channel 17/SAR/ZOH+comparator/Old parallel ZOH comparator ==
  Signal in : Inport
  DAC in : Inport  Port=2
  SAR done : Inport  Port=3
  Clk : Inport  Port=4
  " DAC-signal < delta?" : Subsystem  TreatAsAtomicUnit=on
      mask Display: text(.5, .5, 'Comparator', 'horizontalAlignment', 'center', 'verticalAlignment', 'middle')
  AND : Logic  IconShape=distinctive  AllPortsSameDT=off  OutDataTypeStr=boolean
  AND1 : Logic  IconShape=distinctive  AllPortsSameDT=off  OutDataTypeStr=boolean
  Add : Sum  Inputs=+-
  Constant : Constant  Value=ZOH_delta
  Count ZOH's : Subsystem
  D Latch : simulink_extras/Flip Flops/D Latch
      settings: SourceProductBaseCode=SL
  NOT : Logic  Operator=NOT  IconShape=distinctive  AllPortsSameDT=off  OutDataTypeStr=boolean
  OR : Logic  Operator=OR  IconShape=distinctive  AllPortsSameDT=off  OutDataTypeStr=boolean
  Signal-DAC < delta? : Subsystem  TreatAsAtomicUnit=on
      mask Display: text(.5, .5, 'Comparator', 'horizontalAlignment', 'center', 'verticalAlignment', 'middle')
  Signal>DAC? : Subsystem  TreatAsAtomicUnit=on
      mask Display: text(.5, .5, 'Comparator', 'horizontalAlignment', 'center', 'verticalAlignment', 'middle')
  Subtract : Sum  Inputs=-+
  Comparator_out : Outport
  Output1 : Outport  Port=2
  Output : Outport  Port=3
  wires:
  Signal>DAC?/1(Comparator_out) -> NOT/1, Comparator_out/1, AND1/1
  AND1/1 -> OR/1
  Subtract/1 -> " DAC-signal < delta?"/2(DAC_in)
  Signal in/1 -> Add/1, Subtract/1, Signal>DAC?/1(y(t))
  Clk/1 -> Signal>DAC?/Trigger, Signal-DAC < delta?/Trigger, " DAC-signal < delta?"/Trigger
  AND/1 -> OR/2
  " DAC-signal < delta?"/1(Comparator_out) -> AND/2  "comp2"
  Signal-DAC < delta?/1(Comparator_out) -> AND1/2  "comp1"
  Add/1 -> Signal-DAC < delta?/2(DAC_in)
  DAC in/1 -> Subtract/2, Add/2, Signal>DAC?/2(DAC_in)
  Constant/1 -> Signal-DAC < delta?/1(y(t)), " DAC-signal < delta?"/1(y(t))
  NOT/1 -> AND/1
  OR/1 -> D Latch/1
  D Latch/1 -> Count ZOH's/1(In1), Output1/1
  Count ZOH's/1(Out1) -> Output/1
  SAR done/1 -> Count ZOH's/Trigger, D Latch/2

== system MMADC/Sensing Channel 18/SAR/ZOH+comparator/Comparator ==
  y(t) : Inport
  DAC_in : Inport  Port=2
  Add : Sum
  Add1 : Sum
  Compare To Zero : simulink/Logic and Bit Operations/Compare To Zero  relop=>  OutDataTypeStr=boolean
  Constant : Constant  Value=comparator_high_offset
  Constant1 : Constant  Value=comparator_low_offset
  Constant2 : Constant  Value=0
  Constant3 : Constant  Value=comparator_offset_on
  Constant4 : Constant  Value=0
  Constant5 : Constant  Value=comparator_noise_on
  Multiply : Gain  Gain=comparator_noise_rms
  Random Number : RandomNumber  SampleTime=1/clk_freq
  Subtract : Sum  Inputs=+-
  Switch : Switch  Criteria=u2 > Threshold
  Switch1 : Switch  Criteria=u2 > Threshold
  Switch2 : Switch  Criteria=u2 > Threshold
  Unit Delay : UnitDelay  SampleTime=-1  HasFrameUpgradeWarning=on
  Comparator_out : Outport
  wires:
  Switch/1 -> Switch1/1
  Subtract/1 -> Add/1
  Constant/1 -> Switch/1
  Constant2/1 -> Switch1/3
  Add/1 -> Compare To Zero/1
  Switch1/1 -> Add/2
  Constant3/1 -> Switch1/2
  Unit Delay/1 -> Switch/2
  Constant1/1 -> Switch/3
  DAC_in/1 -> Subtract/2
  Add1/1 -> Subtract/1
  y(t)/1 -> Add1/2
  Random Number/1 -> Multiply/1
  Switch2/1 -> Add1/1
  Multiply/1 -> Switch2/1
  Constant4/1 -> Switch2/3
  Constant5/1 -> Switch2/2
  Compare To Zero/1 -> Unit Delay/1, Comparator_out/1

== system MMADC/Sensing Channel 18/SAR/ZOH+comparator/Count ZOH's ==
  Trigger : TriggerPort  VariantControl=Variant  PortDimensions=1
  Add : Sum  AccumDataTypeStr=double  OutDataTypeStr=double
  Constant : Constant
  Unit Delay : UnitDelay  SampleTime=-1  HasFrameUpgradeWarning=on
  Out1 : Outport
  wires:
  Constant/1 -> Add/1
  Add/1 -> Unit Delay/1, Out1/1
  Unit Delay/1 -> Add/2
